simulink model "Windturbine"  (Simulink 7.2)
settings: Solver=ode3  StartTime=0  StopTime=30  FixedStep=1  MaxStep=0.2  RelTol=1e-3
values from neighbouring files (symbols this model uses):
  Cp_factor_wind = t.Cp_factor_wind    [wind_ini.m]
  el_power = t.el_power    [wind_ini.m]
  hub_height = t.hub_height    [wind_ini.m]
  rotor_diameter = t.rotor_diameter    [wind_ini.m]
libraries: simulink x1
settings Model: Creator=reisenberger  LastModifiedBy=Reisenberger

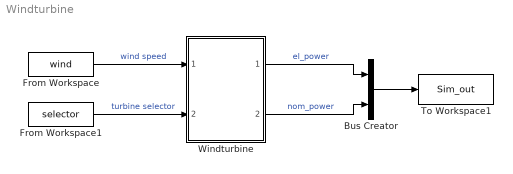
== system Windturbine ==
  Bus Creator : BusCreator  Inputs=2
  From Workspace : FromWorkspace  VariableName=wind  SampleTime=0  OutputAfterFinalValue=Setting to zero
  From Workspace1 : FromWorkspace  VariableName=selector  SampleTime=0  OutputAfterFinalValue=Setting to zero
  To Workspace1 : ToWorkspace  VariableName=Sim_out  SampleTime=-1  SaveFormat=Structure With Time
  Windturbine : Subsystem  mask{v_stop=25, rho=1.225, alpha_hell=0.16, h_ref=10, DisplayTurbChar=off}
      mask prompts: v_stop "Abschaltwindgeschwindigkeit (m/s)"; rho "Luftdichte (kg/m^3)"; alpha_hell "Rauhigkeitsexponent"; h_ref "Referenzhöhe für Höhenformel (m)"; DisplayTurbChar "Display wind turbine power characteristics"
      mask init:
      | %Wind turbine typical characteristic data
      | %c2=116;c3=0.4;c4=5;c5=21;
      | %Computation of c1 and c6 for lambda_nom et cpmax
      | %lambda_nom=8.1;
      | %cp_max=0.48;
      | %cp_nom=cp_max;
      | 
      | %lambda_i_nom=1/(1/lambda_nom-0.035);
      | %k_nom=-(c2*c5/lambda_i_nom-c4*c5-c2)*exp(-c5/lambda_i_nom)/lambda_nom^2;
      | %c1=cp_max/((c2/lambda_i_nom-c4)*exp(-c5/lambda_i_nom)+k_nom*lambda_nom);
      | %c6=k_nom*c1;
      | power_initmask();
      mask CallbackString:
      | ||||DisplayTurbChar=get_param(gcb,'DisplayTurbChar');
      | 
      | if strcmp(DisplayTurbChar,'on')
      |     fig_num=figure;
      | 	clf(fig_num);
      | 	[v_start,v_nom,v_stop,P_nom]=getSPSmaskvalues(gcb,{'v_start','v_nom','v_stop','P_nom'});
      | 
      |     wind_speed = linspace(0,30,300)';
      |     power = ones(length(wind_speed), 1);
      |     for k=1:length(wind_speed)
      |        if wind_speed(k,1) > v_stop
      |            power(k,1) = 0;
      |            %break;
      |        elseif wind_speed(k,1) > v_nom
      |            power(k,1) = P_nom;
      |            %break;
      |        elseif wind_speed(k,1) > v_start
      |            power(k,1) = P_nom*wind_speed(k,1)^3/v_nom^3*(1+v_start^3/v_nom^3) - P_nom*v_start^3/v_nom^3;
      |            %break;
      |        else
      |            power(k,1) = 0;
      |        end
      |     end
      | 
      | 
      |     plot(wind_speed, power);
      |     xlabel('Wind speed (m/s)')
      |     ylabel('Turbine output power (kW)')
      |     title(sprintf('Turbine Power Characteristics (Nominal Power = %0.4g kW)',P_nom))
      |     set_param(gcb,'DisplayTurbChar','off')
      | end
      mask Display: image(imread('Wind.jpg'))
  wires:
  From Workspace/1 -> Windturbine/1(wind_speed)  "wind speed"
  Windturbine/1(el_Power) -> Bus Creator/1  "el_power"
  Windturbine/2(nom_el_Power) -> Bus Creator/2  "nom_power"
  Bus Creator/1 -> To Workspace1/1
  From Workspace1/1 -> Windturbine/2(turbine_selector)  "turbine selector"

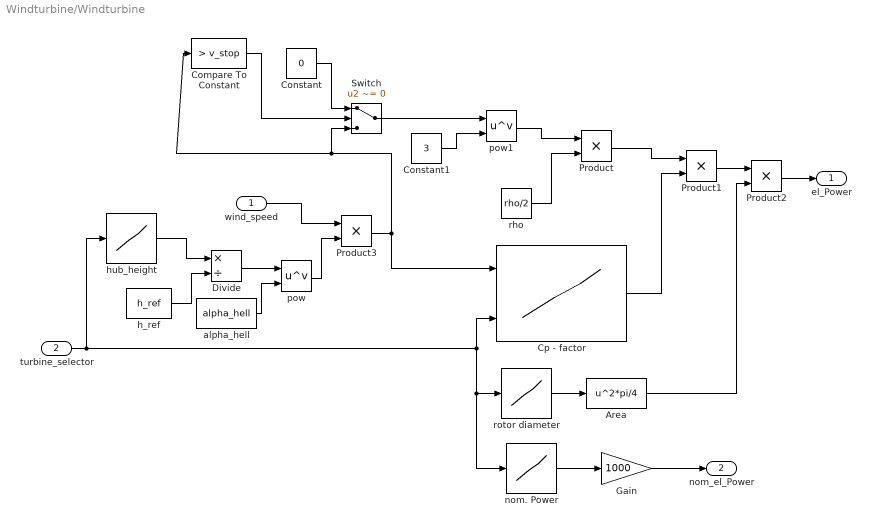
== system Windturbine/Windturbine ==
  wind_speed : Inport  OutDataType=sfix(16)  OutScaling=2^0
  turbine_selector : Inport  Port=2  OutDataType=sfix(16)  OutScaling=2^0
  Area : Fcn  Expr=u^2*pi/4
  Compare To Constant : simulink/Logic and Bit Operations/Compare To Constant  SystemSampleTime=-1  relop=>  const=v_stop  LogicOutDataTypeMode=uint8  ZeroCross=off
  Constant : Constant  Value=0  OutDataType=sfix(16)  OutScaling=2^0
  Constant1 : Constant  Value=3  OutDataType=sfix(16)  OutScaling=2^0
  Cp - factor : Lookup2D  LoadFcn=wind_ini  InitFcn=wind_ini  StartFcn=wind_ini  RowIndex=[0:25]  ColumnIndex=[1:6]  Table=Cp_factor_wind  OutDataType=sfix(16)  OutScaling=2^0
  Divide : Product  Inputs=*/  OutDataType=sfix(16)  OutScaling=2^-10
  Gain : Gain  Gain=1000  ParameterDataType=sfix(16)  ParameterScaling=2^0  OutDataType=sfix(16)  OutScaling=2^0
  Product{,1..3} (4 alike) : Product  OutDataType=sfix(16)  OutScaling=2^0  RndMeth=Zero
  Switch : Switch  Criteria=u2 ~= 0  OutDataType=sfix(16)  OutScaling=2^0
  alpha_hell : Constant  Value=alpha_hell  OutDataType=sfix(16)  OutScaling=2^0
  h_ref : Constant  Value=h_ref  OutDataType=sfix(16)  OutScaling=2^0
  hub_height : Lookup  InputValues=[1:6]  Table=hub_height  OutDataType=sfix(16)  OutScaling=2^0
  nom. Power : Lookup  InputValues=[1:6]  Table=el_power  OutDataType=sfix(16)  OutScaling=2^0
  pow : Math  Operator=pow  OutDataType=sfix(16)  OutScaling=2^0  SaturateOnIntegerOverflow=on
  pow1 : Math  Operator=pow  OutDataType=sfix(16)  OutScaling=2^0  SaturateOnIntegerOverflow=on
  rho : Constant  Value=rho/2  OutDataType=sfix(16)  OutScaling=2^0
  rotor diameter : Lookup  InputValues=[1:6]  Table=rotor_diameter  OutDataType=sfix(16)  OutScaling=2^0
  el_Power : Outport  OutDataType=sfix(16)  OutScaling=2^0
  nom_el_Power : Outport  Port=2  OutDataType=sfix(16)  OutScaling=2^0
  wires:
  Compare To Constant/1 -> Switch/2
  Constant/1 -> Switch/1
  Switch/1 -> pow1/1
  Constant1/1 -> pow1/2
  pow1/1 -> Product/1
  rho/1 -> Product/2
  turbine_selector/1 -> Cp - factor/2, rotor diameter/1, nom. Power/1, hub_height/1
  Product/1 -> Product1/1
  Cp - factor/1 -> Product1/2
  rotor diameter/1 -> Area/1
  Product1/1 -> Product2/1
  Area/1 -> Product2/2
  nom. Power/1 -> Gain/1
  Product2/1 -> el_Power/1
  Gain/1 -> nom_el_Power/1
  hub_height/1 -> Divide/1
  h_ref/1 -> Divide/2
  Divide/1 -> pow/1
  alpha_hell/1 -> pow/2
  wind_speed/1 -> Product3/1
  pow/1 -> Product3/2
  Product3/1 -> Compare To Constant/1, Switch/3, Cp - factor/1
